simulink model "Buck"  (R2022b)
settings: Solver=VariableStepAuto  StartTime=0.0  StopTime=0.05  RelTol=1e-3
values from neighbouring files (symbols this model uses):
  C = 10e-6    (= 1e-05)    [convertidor.m]    (also in variables.m)
  L = 2e-3    (= 0.002)    [convertidor.m]    (also in variables.m)
  R = 10    [convertidor.m]    (also in variables.m)
  U = 32    [convertidor.m]    (also in variables.m)
settings Model: Creator=nemesis  LastModifiedBy=nemesis

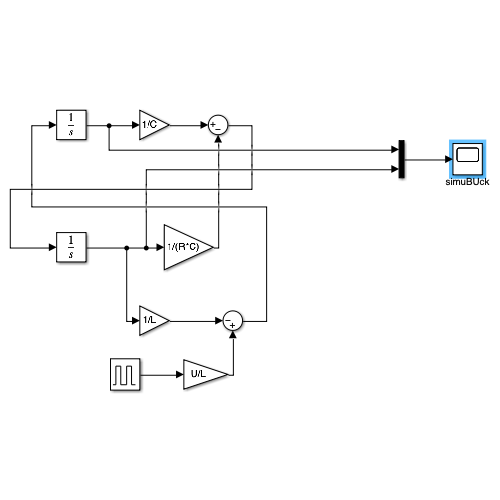
[thumbnail: Simulink's stored preview of the top-level diagram]
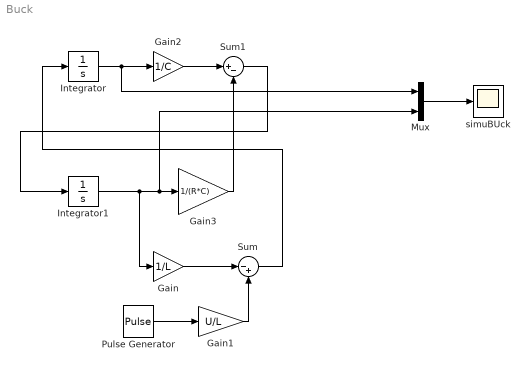
== system Buck ==
  Gain : Gain  Gain=1/L
  Gain1 : Gain  Gain=U/L
  Gain2 : Gain  Gain=1/C
  Gain3 : Gain  Gain=1/(R*C)
  Integrator : Integrator
  Integrator1 : Integrator
  Mux : Mux  Inputs=2
  Pulse Generator : DiscretePulseGenerator  PulseType=Time based  Period=0.00001  PulseWidth=40
  Sum : Sum  Inputs=|-+
  Sum1 : Sum  Inputs=|+-
  simuBUck : Scope
  wires:
  Integrator1/1 -> Gain/1, Mux/2, Gain3/1
  Gain1/1 -> Sum/2
  Pulse Generator/1 -> Gain1/1
  Sum/1 -> Integrator/1
  Gain/1 -> Sum/1
  Integrator/1 -> Mux/1, Gain2/1
  Gain2/1 -> Sum1/1
  Gain3/1 -> Sum1/2
  Sum1/1 -> Integrator1/1
  Mux/1 -> simuBUck/1
